simulink model "DiMauro_Galluzzi_Andres_2024_finalversion"  (R2024a)
settings: Solver=VariableStepAuto  StartTime=0.0  StopTime=simulation_time  RelTol=1e-3
values from neighbouring files (symbols this model uses):
  Ap = zeros(3)    [main.m]
  Bp = eye(3)    [main.m]
  degrad_flag = 1    [main.m]
  F = [e e e e e e; F_low]    [main.m]
  f_ex = 1    [main.m]
  g = 9.81    [main.m]
  Gamma_a = 0.001*eye(6)    [main.m]
  inv_M_tot = inv(M_tot)    [main.m]
  k_f = 3.65e-6    (= 3.65e-06)    [main.m]
  k_i_pos_control = K(3)    [main.m]
  k_omega = diag([K_w_x,K_w_y,K_w_z])    [main.m]
  k_p_pos_control = K(1)    [main.m]
  k_v_pos_control = K(2)    [main.m]
  L = 1    [main.m]
  lambda_r_0 = lambda_r*ones(6,1)    [main.m]
  M_tot = UAV.M+M_box    [main.m]
  omega_cmd_trim_1 = sqrt(UAV.m*g/(UAV.Nr*k_f))*[1 1 1 1 1 1]'    [main.m]
  omega_cmd_trim_2 = sqrt(T_rotor/k_f)*[1 1 1 1 1 1]'    [main.m]
  omega_r_0 = omega_cmd_trim_2    [main.m]
  omega_t = 0.1    [main.m]
  omegab_0 = [0 0 0]'    [main.m]
  p_0 = [0 0 1]'    [main.m]
  pert = 0*[1 1 1 0 0 0]'    [main.m]
  q_0 = eul2quat([0,theta_trim_2,0],'ZYX')'    [main.m]
  radius = 4    [main.m]
  t_pert = 50    [main.m]
  traj = 5    [main.m]
  trim_flag = 0    [main.m]
  vb_0 = 2*[cos(theta_trim_2) 0 sin(theta_trim_2)]'    [main.m]
  w_t = 1    [main.m]
undefined symbols (not defined in the file or in its folder): k_d_pos, k_i_velocity_control, UAV
libraries: slpidlib x6
settings Model: Creator=matti  LastModifiedBy=matti

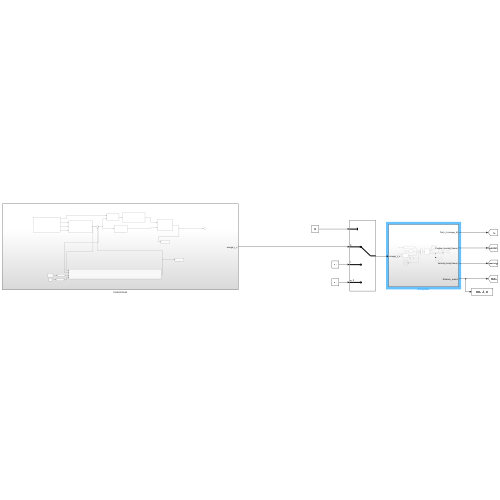
[thumbnail: Simulink's stored preview of the top-level diagram]
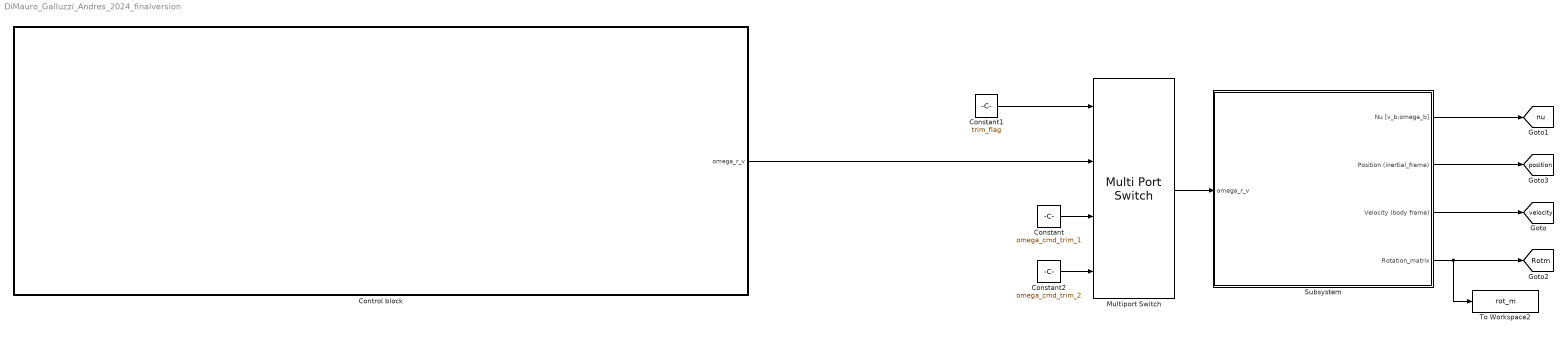
== system DiMauro_Galluzzi_Andres_2024_finalversion ==
  Constant : Constant  Value=omega_cmd_trim_1
  Constant1 : Constant  Value=trim_flag
  Constant2 : Constant  Value=omega_cmd_trim_2
  Control block : Subsystem
  Multiport Switch : MultiPortSwitch  DataPortOrder=Zero-based contiguous  zeroidx=on  SaturateOnIntegerOverflow=off  InputSameDT=off
  Subsystem : Subsystem
  To Workspace2 : ToWorkspace  VariableName=rot_m  SaveFormat=Timeseries  SampleTime=-1
  tag scope: Rotm=global, nu=global, position=global, velocity=global
  wires:
  Subsystem/1(Nu [v_b;omega_b]) -> [nu]
  Constant/1 -> Multiport Switch/3
  Constant2/1 -> Multiport Switch/4
  Subsystem/2(Position (inertial_frame)) -> [position]
  Subsystem/4(Rotation_matrix) -> To Workspace2/1, [Rotm]
  Subsystem/3(Velocity (body frame)) -> [velocity]
  Constant1/1 -> Multiport Switch/1
  Control block/1(omega_r_v) -> Multiport Switch/2
  Multiport Switch/1 -> Subsystem/1(omega_r_v)

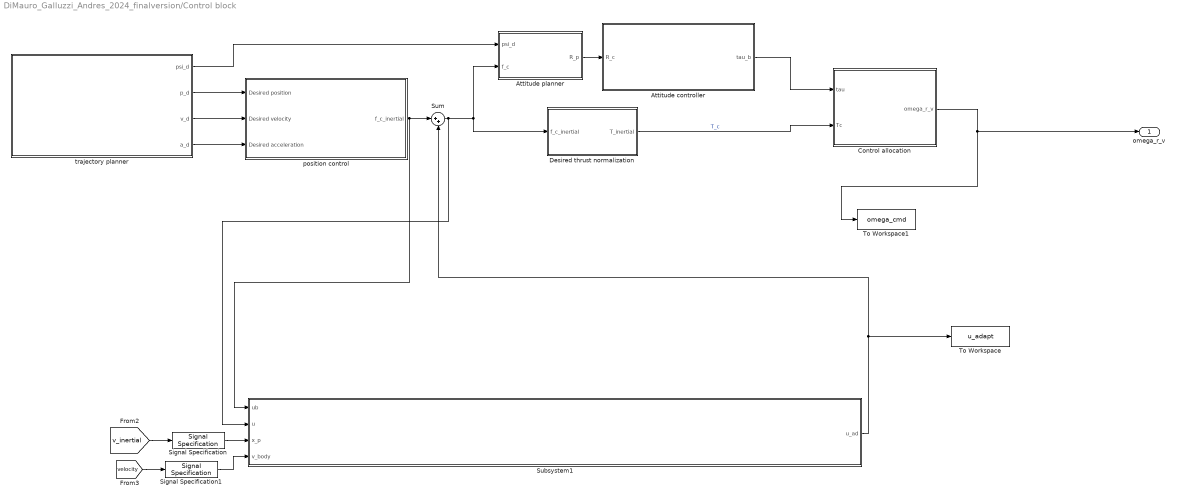
== system DiMauro_Galluzzi_Andres_2024_finalversion/Control block ==
  Attitude controller : Subsystem
  Attitude planner : MATLAB Function  TreatAsAtomicUnit=on
  Control allocation : MATLAB Function  TreatAsAtomicUnit=on
  Desired thrust normalization : MATLAB Function  TreatAsAtomicUnit=on
  Signal Specification : SignalSpecification  Dimensions=3
  Signal Specification1 : SignalSpecification  Dimensions=3
  Subsystem1 : Subsystem  Variant=on  AllowZeroVariantControls=on
  Sum : Sum  Inputs=|++
  To Workspace : ToWorkspace  VariableName=u_adapt  SaveFormat=Timeseries  SampleTime=-1
  To Workspace1 : ToWorkspace  VariableName=omega_cmd  SaveFormat=Timeseries  SampleTime=-1
  position control : Subsystem
  "trajectory planner " : Subsystem
  omega_r_v : Outport
  wires:
  Signal Specification/1 -> Subsystem1/3(x_p)
  Control allocation/1(omega_r_v) -> omega_r_v/1, To Workspace1/1
  Sum/1 -> Desired thrust normalization/1(f_c_inertial), Attitude planner/2(f_c), Subsystem1/2(u)
  Attitude planner/1(R_p) -> Attitude controller/1(R_c)
  [velocity] -> Signal Specification1/1
  Signal Specification1/1 -> Subsystem1/4(v_body)
  "trajectory planner "/1(psi_d) -> Attitude planner/1(psi_d)
  "trajectory planner "/2(p_d) -> position control/1(Desired position)
  [v_inertial] -> Signal Specification/1
  "trajectory planner "/3(v_d) -> position control/2(Desired velocity)
  Subsystem1/1(u_ad) -> To Workspace/1, Sum/2
  Desired thrust normalization/1(T_inertial) -> Control allocation/2(Tc)  "T_c"
  Attitude controller/1(tau_b) -> Control allocation/1(tau)
  "trajectory planner "/4(a_d) -> position control/3(Desired acceleration)
  position control/1(f_c_inertial) -> Sum/1, Subsystem1/1(ub)

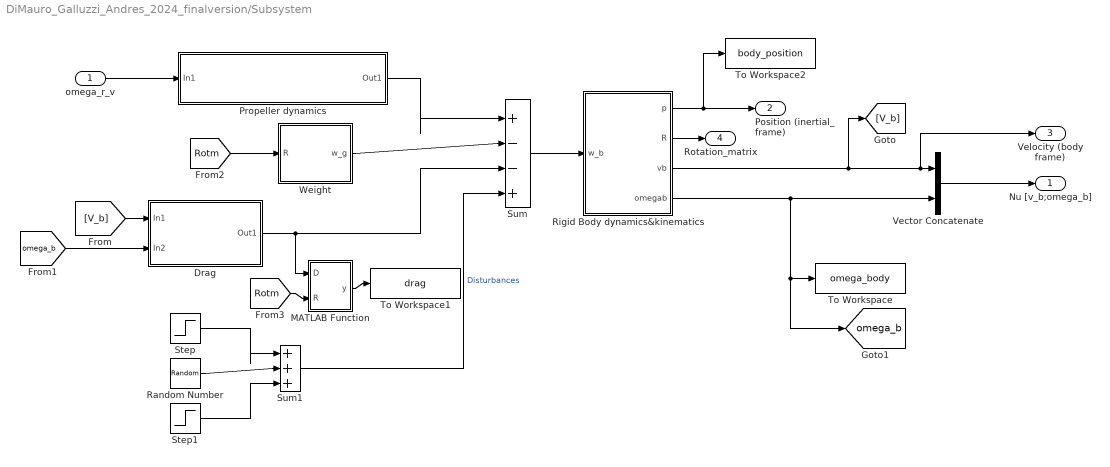
== system DiMauro_Galluzzi_Andres_2024_finalversion/Subsystem ==
  omega_r_v : Inport
  Drag : Subsystem
  MATLAB Function : MATLAB Function  TreatAsAtomicUnit=on
  Propeller dynamics : Subsystem
  Random Number : RandomNumber  Mean=[0 0 0 0 0 0]'  Variance=f_ex/20*[1 1 1 0 0 0]'  SampleTime=0.1
  "Rigid Body dynamics&kinematics " : Subsystem
  Step : Step  Time=t_pert  Before=0*[1 1 1 0 0 0]';  After=f_ex*[1 1 1 0 0 0]';  SampleTime=0
  Step1 : Step  Time=t_pert+5  Before=0*[1 1 1 0 0 0]';  After=-f_ex*[1 1 1 0 0 0]';  SampleTime=0
  Sum : Sum  Inputs=|+--+
  Sum1 : Sum  Inputs=|+++
  To Workspace : ToWorkspace  VariableName=omega_body  SaveFormat=Timeseries  SampleTime=-1
  To Workspace1 : ToWorkspace  VariableName=drag  SaveFormat=Timeseries  SampleTime=-1
  To Workspace2 : ToWorkspace  VariableName=body_position  SaveFormat=Timeseries  SampleTime=-1
  Vector Concatenate : Concatenate
  Weight : MATLAB Function  TreatAsAtomicUnit=on
  Nu [v_b;omega_b] : Outport
  Position (inertial_frame) : Outport  Port=2
  Velocity (body frame) : Outport  Port=3
  Rotation_matrix : Outport  Port=4
  tag scope: omega_b=global
  wires:
  "Rigid Body dynamics&kinematics "/3(vb) -> [V_b], Velocity (body frame)/1, Vector Concatenate/1
  [V_b] -> Drag/1(In1)
  "Rigid Body dynamics&kinematics "/4(omegab) -> [omega_b], To Workspace/1, Vector Concatenate/2
  Propeller dynamics/1(Out1) -> Sum/1
  Weight/1(w_g) -> Sum/2
  [Rotm] -> Weight/1(R)
  [omega_b] -> Drag/2(In2)
  Sum/1 -> "Rigid Body dynamics&kinematics "/1(w_b)
  omega_r_v/1 -> Propeller dynamics/1(In1)
  Vector Concatenate/1 -> Nu [v_b;omega_b]/1
  "Rigid Body dynamics&kinematics "/1(p) -> To Workspace2/1, Position (inertial_frame)/1
  "Rigid Body dynamics&kinematics "/2(R) -> Rotation_matrix/1
  Drag/1(Out1) -> MATLAB Function/1(D), Sum/3
  Random Number/1 -> Sum1/2
  Sum1/1 -> Sum/4  "Disturbances"
  Step/1 -> Sum1/1
  Step1/1 -> Sum1/3
  MATLAB Function/1(y) -> To Workspace1/1
  [Rotm] -> MATLAB Function/2(R)

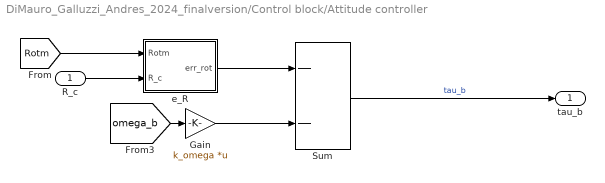
== system DiMauro_Galluzzi_Andres_2024_finalversion/Control block/Attitude controller ==
  R_c : Inport
  Gain : Gain  Gain=k_omega  Multiplication=Matrix(K*u)
  Sum : Sum  Inputs=--
  e_R : MATLAB Function  TreatAsAtomicUnit=on
  tau_b : Outport
  wires:
  e_R/1(err_rot) -> Sum/1
  [Rotm] -> e_R/1(Rotm)
  Sum/1 -> tau_b/1  "tau_b"
  [omega_b] -> Gain/1
  R_c/1 -> e_R/2(R_c)
  Gain/1 -> Sum/2

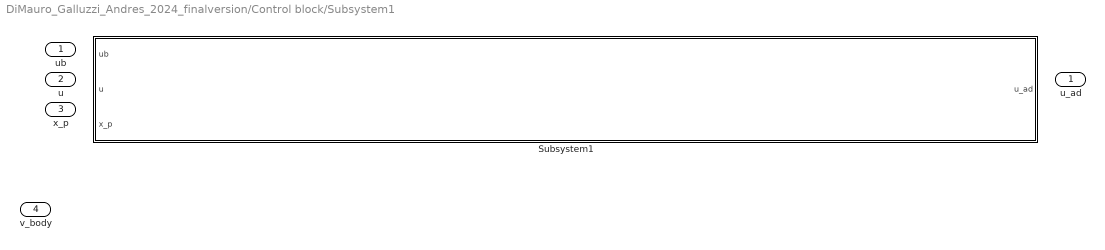
== system DiMauro_Galluzzi_Andres_2024_finalversion/Control block/Subsystem1 ==
  ub : Inport
  u : Inport  Port=2
  x_p : Inport  Port=3
  v_body : Inport  Port=4
  Subsystem1 : Subsystem  VariantControl=flag_adaptive==1
  u_ad : Outport

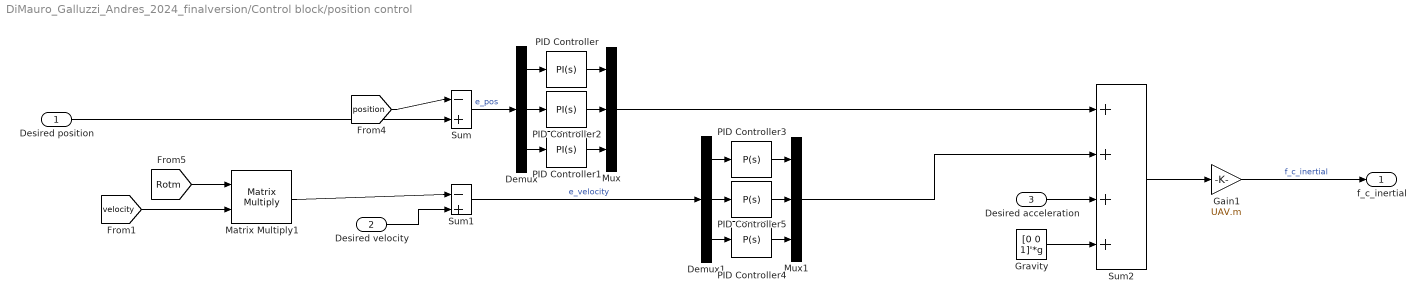
== system DiMauro_Galluzzi_Andres_2024_finalversion/Control block/position control ==
  Desired position : Inport
  Desired velocity : Inport  Port=2
  Desired acceleration : Inport  Port=3
  Demux : Demux  Outputs=3
  Demux1 : Demux  Outputs=3
  Gain1 : Gain  Gain=UAV.m
  Gravity : Constant  Value=[0 0 1]'*g
  Matrix Multiply1 : Product  Multiplication=Matrix(*)
  Mux : Mux  Inputs=3
  Mux1 : Mux  Inputs=3
  PID Controller : slpidlib/PID Controller  Controller=PI  Form=Parallel  TimeDomain=Continuous-time  UseExternalTs=off  SampleTime=-1  IntegratorMethod=Forward Euler  FilterMethod=Forward Euler  ControllerParametersSource=internal  P=k_p_pos_control  I=k_i_pos_control  UseKiTs=off  D=k_d_pos  UseExternalDerivativeSource=off  N=100  UseFilter=on  TunerSelectOption=Transfer Function Based (PID Tuner App)  InitialConditionSource=internal  InitialConditionForIntegrator=0  InitialConditionForFilter=0  DifferentiatorICPrevScaledInput=0  ExternalReset=none  TrackingMode=off  Kt=1  LimitOutput=off  SatLimitsSource=internal  UpperSaturationLimit=inf  LowerSaturationLimit=-inf  LinearizeAsGain=on  AntiWindupMode=none  Kb=1  LimitIntegrator=off  UpperIntegratorSaturationLimit=inf  LowerIntegratorSaturationLimit=-inf  POutMin=[]  POutMax=[]  IOutMin=[]  IOutMax=[]  DOutMin=[]  DOutMax=[]  NOutMin=[]  NOutMax=[]  SumOutMin=[]  SumOutMax=[]  SaturationOutMin=[]  SaturationOutMax=[]  PParamMin=[]  PParamMax=[]  IParamMin=[]  IParamMax=[]  DParamMin=[]  DParamMax=[]  NParamMin=[]  NParamMax=[]  KbParamMin=[]  KbParamMax=[]  KtParamMin=[]  KtParamMax=[]  KbOutMin=[]  KbOutMax=[]  KtOutMin=[]  KtOutMax=[]  IntegratorOutMin=[]  IntegratorOutMax=[]  FilterOutMin=[]  FilterOutMax=[]  SumI1OutMin=[]  SumI1OutMax=[]  SumI2OutMin=[]  SumI2OutMax=[]  SumI3OutMin=[]  SumI3OutMax=[]  SumI4OutMin=[]  SumI4OutMax=[]  SumDOutMin=[]  SumDOutMax=[]  DifferentiatorOutMin=[]  DifferentiatorOutMax=[]  FilterDiffOutCoefMin=[]  FilterDiffOutCoefMax=[]  ReciprocalOutMin=[]  ReciprocalOutMax=[]  SumDenOutMin=[]  SumDenOutMax=[]  SumNumOutMin=[]  SumNumOutMax=[]  DivideOutMin=[]  DivideOutMax=[]  UdiffTsProdOutMin=[]  UdiffTsProdOutMax=[]  NTsProdOutMin=[]  NTsProdOutMax=[]  UintegralTsProdOutMin=[]  UintegralTsProdOutMax=[]  UngainTsProdOutMin=[]  UngainTsProdOutMax=[]  ClampingZeroOutDataTypeStr=Inherit: Inherit via back propagation  ClampingZeroOutMin=[]  ClampingZeroOutMax=[]  FilterDenConstantOutDataTypeStr=Inherit: Inherit via back propagation  FilterDenConstantOutMin=[]  FilterDenConstantOutMax=[]  PCopyOutDataTypeStr=Inherit: Inherit via back propagation  PCopyOutMin=[]  PCopyOutMax=[]  NCopyOutDataTypeStr=Inherit: Inherit via back propagation  NCopyOutMin=[]  NCopyOutMax=[]  IntegratorContinuousStateAttributes=''  IntegratorStateMustResolveToSignalObject=off  IntegratorRTWStateStorageClass=Auto  FilterContinuousStateAttributes=''  FilterStateMustResolveToSignalObject=off  FilterRTWStateStorageClass=Auto  ParallelPVariant=InternalParameters  IdealPVariant=Disabled  IVariant=InternalParameters  DVariant=Disabled  IntegratorVariant=Continuous  SatVariant=Disabled  AWVariant=Passthrough  PCopyVariant=Disabled  TRVariant=Disabled  FdbkBlocksVariant=Forward  IdealPFdbkVariant=Disabled  SatFdbkVariant=Disabled  DerivativeFilterVariant=Disabled  NVariant=Disabled  NCopyVariant=Disabled_SignalSpec  FilterICVariant=Disabled  IntegratorICVariant=InternalICs  ExternalResetVariant=Disabled  TRSumVariant=Passthrough  SumFdbkVariant=Disabled  SumVariant=Sum_PI  TsampFilterVariant=InternalTs  TsampNgainVariant=Passthrough  TsampIntegralVariant=Disabled_SignalSpec  ExternalSaturationOutDataTypeStr=Inherit: Same as second input  DerivativeSourceVariant=Disabled
  PID Controller1 : slpidlib/PID Controller  Controller=PI  Form=Parallel  TimeDomain=Continuous-time  UseExternalTs=off  SampleTime=-1  IntegratorMethod=Forward Euler  FilterMethod=Forward Euler  ControllerParametersSource=internal  P=k_p_pos_control  I=k_i_pos_control  UseKiTs=off  D=k_d_pos  UseExternalDerivativeSource=off  N=100  UseFilter=on  TunerSelectOption=Transfer Function Based (PID Tuner App)  InitialConditionSource=internal  InitialConditionForIntegrator=0  InitialConditionForFilter=0  DifferentiatorICPrevScaledInput=0  ExternalReset=none  TrackingMode=off  Kt=1  LimitOutput=off  SatLimitsSource=internal  UpperSaturationLimit=inf  LowerSaturationLimit=-inf  LinearizeAsGain=on  AntiWindupMode=none  Kb=1  LimitIntegrator=off  UpperIntegratorSaturationLimit=inf  LowerIntegratorSaturationLimit=-inf  POutMin=[]  POutMax=[]  IOutMin=[]  IOutMax=[]  DOutMin=[]  DOutMax=[]  NOutMin=[]  NOutMax=[]  SumOutMin=[]  SumOutMax=[]  SaturationOutMin=[]  SaturationOutMax=[]  PParamMin=[]  PParamMax=[]  IParamMin=[]  IParamMax=[]  DParamMin=[]  DParamMax=[]  NParamMin=[]  NParamMax=[]  KbParamMin=[]  KbParamMax=[]  KtParamMin=[]  KtParamMax=[]  KbOutMin=[]  KbOutMax=[]  KtOutMin=[]  KtOutMax=[]  IntegratorOutMin=[]  IntegratorOutMax=[]  FilterOutMin=[]  FilterOutMax=[]  SumI1OutMin=[]  SumI1OutMax=[]  SumI2OutMin=[]  SumI2OutMax=[]  SumI3OutMin=[]  SumI3OutMax=[]  SumI4OutMin=[]  SumI4OutMax=[]  SumDOutMin=[]  SumDOutMax=[]  DifferentiatorOutMin=[]  DifferentiatorOutMax=[]  FilterDiffOutCoefMin=[]  FilterDiffOutCoefMax=[]  ReciprocalOutMin=[]  ReciprocalOutMax=[]  SumDenOutMin=[]  SumDenOutMax=[]  SumNumOutMin=[]  SumNumOutMax=[]  DivideOutMin=[]  DivideOutMax=[]  UdiffTsProdOutMin=[]  UdiffTsProdOutMax=[]  NTsProdOutMin=[]  NTsProdOutMax=[]  UintegralTsProdOutMin=[]  UintegralTsProdOutMax=[]  UngainTsProdOutMin=[]  UngainTsProdOutMax=[]  ClampingZeroOutDataTypeStr=Inherit: Inherit via back propagation  ClampingZeroOutMin=[]  ClampingZeroOutMax=[]  FilterDenConstantOutDataTypeStr=Inherit: Inherit via back propagation  FilterDenConstantOutMin=[]  FilterDenConstantOutMax=[]  PCopyOutDataTypeStr=Inherit: Inherit via back propagation  PCopyOutMin=[]  PCopyOutMax=[]  NCopyOutDataTypeStr=Inherit: Inherit via back propagation  NCopyOutMin=[]  NCopyOutMax=[]  IntegratorContinuousStateAttributes=''  IntegratorStateMustResolveToSignalObject=off  IntegratorRTWStateStorageClass=Auto  FilterContinuousStateAttributes=''  FilterStateMustResolveToSignalObject=off  FilterRTWStateStorageClass=Auto  ParallelPVariant=InternalParameters  IdealPVariant=Disabled  IVariant=InternalParameters  DVariant=Disabled  IntegratorVariant=Continuous  SatVariant=Disabled  AWVariant=Passthrough  PCopyVariant=Disabled  TRVariant=Disabled  FdbkBlocksVariant=Forward  IdealPFdbkVariant=Disabled  SatFdbkVariant=Disabled  DerivativeFilterVariant=Disabled  NVariant=Disabled  NCopyVariant=Disabled_SignalSpec  FilterICVariant=Disabled  IntegratorICVariant=InternalICs  ExternalResetVariant=Disabled  TRSumVariant=Passthrough  SumFdbkVariant=Disabled  SumVariant=Sum_PI  TsampFilterVariant=InternalTs  TsampNgainVariant=Passthrough  TsampIntegralVariant=Disabled_SignalSpec  ExternalSaturationOutDataTypeStr=Inherit: Same as second input  DerivativeSourceVariant=Disabled
  PID Controller2 : slpidlib/PID Controller  Controller=PI  Form=Parallel  TimeDomain=Continuous-time  UseExternalTs=off  SampleTime=-1  IntegratorMethod=Forward Euler  FilterMethod=Forward Euler  ControllerParametersSource=internal  P=k_p_pos_control  I=k_i_pos_control  UseKiTs=off  D=k_d_pos  UseExternalDerivativeSource=off  N=100  UseFilter=on  TunerSelectOption=Transfer Function Based (PID Tuner App)  InitialConditionSource=internal  InitialConditionForIntegrator=0  InitialConditionForFilter=0  DifferentiatorICPrevScaledInput=0  ExternalReset=none  TrackingMode=off  Kt=1  LimitOutput=off  SatLimitsSource=internal  UpperSaturationLimit=inf  LowerSaturationLimit=-inf  LinearizeAsGain=on  AntiWindupMode=none  Kb=1  LimitIntegrator=off  UpperIntegratorSaturationLimit=inf  LowerIntegratorSaturationLimit=-inf  POutMin=[]  POutMax=[]  IOutMin=[]  IOutMax=[]  DOutMin=[]  DOutMax=[]  NOutMin=[]  NOutMax=[]  SumOutMin=[]  SumOutMax=[]  SaturationOutMin=[]  SaturationOutMax=[]  PParamMin=[]  PParamMax=[]  IParamMin=[]  IParamMax=[]  DParamMin=[]  DParamMax=[]  NParamMin=[]  NParamMax=[]  KbParamMin=[]  KbParamMax=[]  KtParamMin=[]  KtParamMax=[]  KbOutMin=[]  KbOutMax=[]  KtOutMin=[]  KtOutMax=[]  IntegratorOutMin=[]  IntegratorOutMax=[]  FilterOutMin=[]  FilterOutMax=[]  SumI1OutMin=[]  SumI1OutMax=[]  SumI2OutMin=[]  SumI2OutMax=[]  SumI3OutMin=[]  SumI3OutMax=[]  SumI4OutMin=[]  SumI4OutMax=[]  SumDOutMin=[]  SumDOutMax=[]  DifferentiatorOutMin=[]  DifferentiatorOutMax=[]  FilterDiffOutCoefMin=[]  FilterDiffOutCoefMax=[]  ReciprocalOutMin=[]  ReciprocalOutMax=[]  SumDenOutMin=[]  SumDenOutMax=[]  SumNumOutMin=[]  SumNumOutMax=[]  DivideOutMin=[]  DivideOutMax=[]  UdiffTsProdOutMin=[]  UdiffTsProdOutMax=[]  NTsProdOutMin=[]  NTsProdOutMax=[]  UintegralTsProdOutMin=[]  UintegralTsProdOutMax=[]  UngainTsProdOutMin=[]  UngainTsProdOutMax=[]  ClampingZeroOutDataTypeStr=Inherit: Inherit via back propagation  ClampingZeroOutMin=[]  ClampingZeroOutMax=[]  FilterDenConstantOutDataTypeStr=Inherit: Inherit via back propagation  FilterDenConstantOutMin=[]  FilterDenConstantOutMax=[]  PCopyOutDataTypeStr=Inherit: Inherit via back propagation  PCopyOutMin=[]  PCopyOutMax=[]  NCopyOutDataTypeStr=Inherit: Inherit via back propagation  NCopyOutMin=[]  NCopyOutMax=[]  IntegratorContinuousStateAttributes=''  IntegratorStateMustResolveToSignalObject=off  IntegratorRTWStateStorageClass=Auto  FilterContinuousStateAttributes=''  FilterStateMustResolveToSignalObject=off  FilterRTWStateStorageClass=Auto  ParallelPVariant=InternalParameters  IdealPVariant=Disabled  IVariant=InternalParameters  DVariant=Disabled  IntegratorVariant=Continuous  SatVariant=Disabled  AWVariant=Passthrough  PCopyVariant=Disabled  TRVariant=Disabled  FdbkBlocksVariant=Forward  IdealPFdbkVariant=Disabled  SatFdbkVariant=Disabled  DerivativeFilterVariant=Disabled  NVariant=Disabled  NCopyVariant=Disabled_SignalSpec  FilterICVariant=Disabled  IntegratorICVariant=InternalICs  ExternalResetVariant=Disabled  TRSumVariant=Passthrough  SumFdbkVariant=Disabled  SumVariant=Sum_PI  TsampFilterVariant=InternalTs  TsampNgainVariant=Passthrough  TsampIntegralVariant=Disabled_SignalSpec  ExternalSaturationOutDataTypeStr=Inherit: Same as second input  DerivativeSourceVariant=Disabled
  PID Controller3 : slpidlib/PID Controller  Controller=P  Form=Parallel  TimeDomain=Continuous-time  UseExternalTs=off  SampleTime=-1  IntegratorMethod=Forward Euler  FilterMethod=Forward Euler  ControllerParametersSource=internal  P=k_v_pos_control  I=k_i_velocity_control  UseKiTs=off  D=0  UseExternalDerivativeSource=off  N=100  UseFilter=on  TunerSelectOption=Transfer Function Based (PID Tuner App)  InitialConditionSource=internal  InitialConditionForIntegrator=0  InitialConditionForFilter=0  DifferentiatorICPrevScaledInput=0  ExternalReset=none  TrackingMode=off  Kt=1  LimitOutput=off  SatLimitsSource=internal  UpperSaturationLimit=inf  LowerSaturationLimit=-inf  LinearizeAsGain=on  AntiWindupMode=none  Kb=1  LimitIntegrator=off  UpperIntegratorSaturationLimit=inf  LowerIntegratorSaturationLimit=-inf  POutMin=[]  POutMax=[]  IOutMin=[]  IOutMax=[]  DOutMin=[]  DOutMax=[]  NOutMin=[]  NOutMax=[]  SumOutMin=[]  SumOutMax=[]  SaturationOutMin=[]  SaturationOutMax=[]  PParamMin=[]  PParamMax=[]  IParamMin=[]  IParamMax=[]  DParamMin=[]  DParamMax=[]  NParamMin=[]  NParamMax=[]  KbParamMin=[]  KbParamMax=[]  KtParamMin=[]  KtParamMax=[]  KbOutMin=[]  KbOutMax=[]  KtOutMin=[]  KtOutMax=[]  IntegratorOutMin=[]  IntegratorOutMax=[]  FilterOutMin=[]  FilterOutMax=[]  SumI1OutMin=[]  SumI1OutMax=[]  SumI2OutMin=[]  SumI2OutMax=[]  SumI3OutMin=[]  SumI3OutMax=[]  SumI4OutMin=[]  SumI4OutMax=[]  SumDOutMin=[]  SumDOutMax=[]  DifferentiatorOutMin=[]  DifferentiatorOutMax=[]  FilterDiffOutCoefMin=[]  FilterDiffOutCoefMax=[]  ReciprocalOutMin=[]  ReciprocalOutMax=[]  SumDenOutMin=[]  SumDenOutMax=[]  SumNumOutMin=[]  SumNumOutMax=[]  DivideOutMin=[]  DivideOutMax=[]  UdiffTsProdOutMin=[]  UdiffTsProdOutMax=[]  NTsProdOutMin=[]  NTsProdOutMax=[]  UintegralTsProdOutMin=[]  UintegralTsProdOutMax=[]  UngainTsProdOutMin=[]  UngainTsProdOutMax=[]  ClampingZeroOutDataTypeStr=Inherit: Inherit via back propagation  ClampingZeroOutMin=[]  ClampingZeroOutMax=[]  FilterDenConstantOutDataTypeStr=Inherit: Inherit via back propagation  FilterDenConstantOutMin=[]  FilterDenConstantOutMax=[]  PCopyOutDataTypeStr=Inherit: Inherit via back propagation  PCopyOutMin=[]  PCopyOutMax=[]  NCopyOutDataTypeStr=Inherit: Inherit via back propagation  NCopyOutMin=[]  NCopyOutMax=[]  IntegratorContinuousStateAttributes=''  IntegratorStateMustResolveToSignalObject=off  IntegratorRTWStateStorageClass=Auto  FilterContinuousStateAttributes=''  FilterStateMustResolveToSignalObject=off  FilterRTWStateStorageClass=Auto  ParallelPVariant=InternalParameters  IdealPVariant=Disabled  IVariant=Disabled  DVariant=Disabled  IntegratorVariant=Disabled  SatVariant=Disabled  AWVariant=Disabled  PCopyVariant=Disabled  TRVariant=Disabled  FdbkBlocksVariant=Forward  IdealPFdbkVariant=Disabled  SatFdbkVariant=Disabled  DerivativeFilterVariant=Disabled  NVariant=Disabled  NCopyVariant=Disabled_SignalSpec  FilterICVariant=Disabled  IntegratorICVariant=Disabled  ExternalResetVariant=Disabled  TRSumVariant=Passthrough  SumFdbkVariant=Disabled  SumVariant=Passthrough_P  TsampFilterVariant=InternalTs  TsampNgainVariant=Passthrough  TsampIntegralVariant=Disabled_SignalSpec  ExternalSaturationOutDataTypeStr=Inherit: Same as second input  DerivativeSourceVariant=Disabled
  PID Controller4 : slpidlib/PID Controller  Controller=P  Form=Parallel  TimeDomain=Continuous-time  UseExternalTs=off  SampleTime=-1  IntegratorMethod=Forward Euler  FilterMethod=Forward Euler  ControllerParametersSource=internal  P=k_v_pos_control  I=k_i_velocity_control*5  UseKiTs=off  D=0  UseExternalDerivativeSource=off  N=100  UseFilter=on  TunerSelectOption=Transfer Function Based (PID Tuner App)  InitialConditionSource=internal  InitialConditionForIntegrator=0  InitialConditionForFilter=0  DifferentiatorICPrevScaledInput=0  ExternalReset=none  TrackingMode=off  Kt=1  LimitOutput=off  SatLimitsSource=internal  UpperSaturationLimit=inf  LowerSaturationLimit=-inf  LinearizeAsGain=on  AntiWindupMode=none  Kb=1  LimitIntegrator=off  UpperIntegratorSaturationLimit=inf  LowerIntegratorSaturationLimit=-inf  POutMin=[]  POutMax=[]  IOutMin=[]  IOutMax=[]  DOutMin=[]  DOutMax=[]  NOutMin=[]  NOutMax=[]  SumOutMin=[]  SumOutMax=[]  SaturationOutMin=[]  SaturationOutMax=[]  PParamMin=[]  PParamMax=[]  IParamMin=[]  IParamMax=[]  DParamMin=[]  DParamMax=[]  NParamMin=[]  NParamMax=[]  KbParamMin=[]  KbParamMax=[]  KtParamMin=[]  KtParamMax=[]  KbOutMin=[]  KbOutMax=[]  KtOutMin=[]  KtOutMax=[]  IntegratorOutMin=[]  IntegratorOutMax=[]  FilterOutMin=[]  FilterOutMax=[]  SumI1OutMin=[]  SumI1OutMax=[]  SumI2OutMin=[]  SumI2OutMax=[]  SumI3OutMin=[]  SumI3OutMax=[]  SumI4OutMin=[]  SumI4OutMax=[]  SumDOutMin=[]  SumDOutMax=[]  DifferentiatorOutMin=[]  DifferentiatorOutMax=[]  FilterDiffOutCoefMin=[]  FilterDiffOutCoefMax=[]  ReciprocalOutMin=[]  ReciprocalOutMax=[]  SumDenOutMin=[]  SumDenOutMax=[]  SumNumOutMin=[]  SumNumOutMax=[]  DivideOutMin=[]  DivideOutMax=[]  UdiffTsProdOutMin=[]  UdiffTsProdOutMax=[]  NTsProdOutMin=[]  NTsProdOutMax=[]  UintegralTsProdOutMin=[]  UintegralTsProdOutMax=[]  UngainTsProdOutMin=[]  UngainTsProdOutMax=[]  ClampingZeroOutDataTypeStr=Inherit: Inherit via back propagation  ClampingZeroOutMin=[]  ClampingZeroOutMax=[]  FilterDenConstantOutDataTypeStr=Inherit: Inherit via back propagation  FilterDenConstantOutMin=[]  FilterDenConstantOutMax=[]  PCopyOutDataTypeStr=Inherit: Inherit via back propagation  PCopyOutMin=[]  PCopyOutMax=[]  NCopyOutDataTypeStr=Inherit: Inherit via back propagation  NCopyOutMin=[]  NCopyOutMax=[]  IntegratorContinuousStateAttributes=''  IntegratorStateMustResolveToSignalObject=off  IntegratorRTWStateStorageClass=Auto  FilterContinuousStateAttributes=''  FilterStateMustResolveToSignalObject=off  FilterRTWStateStorageClass=Auto  ParallelPVariant=InternalParameters  IdealPVariant=Disabled  IVariant=Disabled  DVariant=Disabled  IntegratorVariant=Disabled  SatVariant=Disabled  AWVariant=Disabled  PCopyVariant=Disabled  TRVariant=Disabled  FdbkBlocksVariant=Forward  IdealPFdbkVariant=Disabled  SatFdbkVariant=Disabled  DerivativeFilterVariant=Disabled  NVariant=Disabled  NCopyVariant=Disabled_SignalSpec  FilterICVariant=Disabled  IntegratorICVariant=Disabled  ExternalResetVariant=Disabled  TRSumVariant=Passthrough  SumFdbkVariant=Disabled  SumVariant=Passthrough_P  TsampFilterVariant=InternalTs  TsampNgainVariant=Passthrough  TsampIntegralVariant=Disabled_SignalSpec  ExternalSaturationOutDataTypeStr=Inherit: Same as second input  DerivativeSourceVariant=Disabled
  PID Controller5 : slpidlib/PID Controller  Controller=P  Form=Parallel  TimeDomain=Continuous-time  UseExternalTs=off  SampleTime=-1  IntegratorMethod=Forward Euler  FilterMethod=Forward Euler  ControllerParametersSource=internal  P=k_v_pos_control  I=k_i_velocity_control  UseKiTs=off  D=0  UseExternalDerivativeSource=off  N=100  UseFilter=on  TunerSelectOption=Transfer Function Based (PID Tuner App)  InitialConditionSource=internal  InitialConditionForIntegrator=0  InitialConditionForFilter=0  DifferentiatorICPrevScaledInput=0  ExternalReset=none  TrackingMode=off  Kt=1  LimitOutput=off  SatLimitsSource=internal  UpperSaturationLimit=inf  LowerSaturationLimit=-inf  LinearizeAsGain=on  AntiWindupMode=none  Kb=1  LimitIntegrator=off  UpperIntegratorSaturationLimit=inf  LowerIntegratorSaturationLimit=-inf  POutMin=[]  POutMax=[]  IOutMin=[]  IOutMax=[]  DOutMin=[]  DOutMax=[]  NOutMin=[]  NOutMax=[]  SumOutMin=[]  SumOutMax=[]  SaturationOutMin=[]  SaturationOutMax=[]  PParamMin=[]  PParamMax=[]  IParamMin=[]  IParamMax=[]  DParamMin=[]  DParamMax=[]  NParamMin=[]  NParamMax=[]  KbParamMin=[]  KbParamMax=[]  KtParamMin=[]  KtParamMax=[]  KbOutMin=[]  KbOutMax=[]  KtOutMin=[]  KtOutMax=[]  IntegratorOutMin=[]  IntegratorOutMax=[]  FilterOutMin=[]  FilterOutMax=[]  SumI1OutMin=[]  SumI1OutMax=[]  SumI2OutMin=[]  SumI2OutMax=[]  SumI3OutMin=[]  SumI3OutMax=[]  SumI4OutMin=[]  SumI4OutMax=[]  SumDOutMin=[]  SumDOutMax=[]  DifferentiatorOutMin=[]  DifferentiatorOutMax=[]  FilterDiffOutCoefMin=[]  FilterDiffOutCoefMax=[]  ReciprocalOutMin=[]  ReciprocalOutMax=[]  SumDenOutMin=[]  SumDenOutMax=[]  SumNumOutMin=[]  SumNumOutMax=[]  DivideOutMin=[]  DivideOutMax=[]  UdiffTsProdOutMin=[]  UdiffTsProdOutMax=[]  NTsProdOutMin=[]  NTsProdOutMax=[]  UintegralTsProdOutMin=[]  UintegralTsProdOutMax=[]  UngainTsProdOutMin=[]  UngainTsProdOutMax=[]  ClampingZeroOutDataTypeStr=Inherit: Inherit via back propagation  ClampingZeroOutMin=[]  ClampingZeroOutMax=[]  FilterDenConstantOutDataTypeStr=Inherit: Inherit via back propagation  FilterDenConstantOutMin=[]  FilterDenConstantOutMax=[]  PCopyOutDataTypeStr=Inherit: Inherit via back propagation  PCopyOutMin=[]  PCopyOutMax=[]  NCopyOutDataTypeStr=Inherit: Inherit via back propagation  NCopyOutMin=[]  NCopyOutMax=[]  IntegratorContinuousStateAttributes=''  IntegratorStateMustResolveToSignalObject=off  IntegratorRTWStateStorageClass=Auto  FilterContinuousStateAttributes=''  FilterStateMustResolveToSignalObject=off  FilterRTWStateStorageClass=Auto  ParallelPVariant=InternalParameters  IdealPVariant=Disabled  IVariant=Disabled  DVariant=Disabled  IntegratorVariant=Disabled  SatVariant=Disabled  AWVariant=Disabled  PCopyVariant=Disabled  TRVariant=Disabled  FdbkBlocksVariant=Forward  IdealPFdbkVariant=Disabled  SatFdbkVariant=Disabled  DerivativeFilterVariant=Disabled  NVariant=Disabled  NCopyVariant=Disabled_SignalSpec  FilterICVariant=Disabled  IntegratorICVariant=Disabled  ExternalResetVariant=Disabled  TRSumVariant=Passthrough  SumFdbkVariant=Disabled  SumVariant=Passthrough_P  TsampFilterVariant=InternalTs  TsampNgainVariant=Passthrough  TsampIntegralVariant=Disabled_SignalSpec  ExternalSaturationOutDataTypeStr=Inherit: Same as second input  DerivativeSourceVariant=Disabled
  Sum : Sum  Inputs=|-+
  Sum1 : Sum  Inputs=|-+
  Sum2 : Sum  Inputs=++++
  f_c_inertial : Outport
  wires:
  Sum2/1 -> Gain1/1
  [position] -> Sum/1
  Gravity/1 -> Sum2/4
  Desired velocity/1 -> Sum1/2
  Desired acceleration/1 -> Sum2/3
  Desired position/1 -> Sum/2
  [velocity] -> Matrix Multiply1/2
  Matrix Multiply1/1 -> Sum1/1
  [Rotm] -> Matrix Multiply1/1
  Gain1/1 -> f_c_inertial/1  "f_c_inertial"
  Sum/1 -> Demux/1  "e_pos"
  Demux/2 -> PID Controller2/1
  Demux/3 -> PID Controller1/1
  PID Controller2/1 -> Mux/2
  PID Controller/1 -> Mux/1
  PID Controller1/1 -> Mux/3
  Demux/1 -> PID Controller/1
  Demux1/3 -> PID Controller4/1
  PID Controller3/1 -> Mux1/1
  PID Controller5/1 -> Mux1/2
  PID Controller4/1 -> Mux1/3
  Demux1/2 -> PID Controller5/1
  Demux1/1 -> PID Controller3/1
  Mux1/1 -> Sum2/2
  Sum1/1 -> Demux1/1  "e_velocity"
  Mux/1 -> Sum2/1

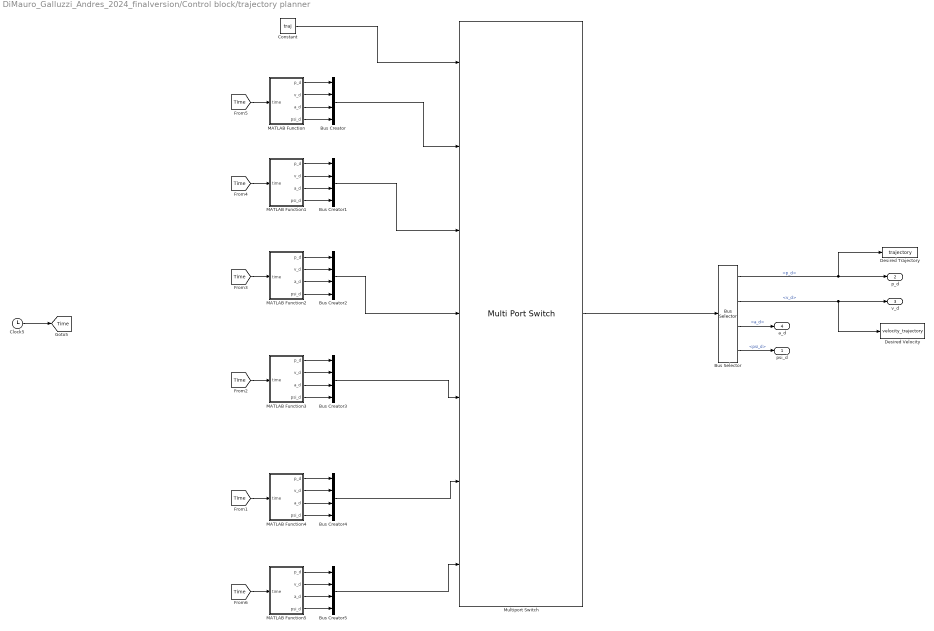
== system DiMauro_Galluzzi_Andres_2024_finalversion/Control block/trajectory planner  ==
  Bus Creator{,1..5} (6 alike) : BusCreator  Inputs=4
  Bus Selector : BusSelector  OutputSignals=p_d,v_d,a_d,psi_d
  Clock5 : Clock
  Constant : Constant  Value=traj
  Desired Trajectory : ToWorkspace  VariableName=trajectory  SaveFormat=Timeseries  SampleTime=-1
  Desired Velocity : ToWorkspace  VariableName=velocity_trajectory  SaveFormat=Timeseries  SampleTime=-1
  MATLAB Function : MATLAB Function  TreatAsAtomicUnit=on
  MATLAB Function1 : MATLAB Function  TreatAsAtomicUnit=on
  MATLAB Function2 : MATLAB Function  TreatAsAtomicUnit=on
  MATLAB Function3 : MATLAB Function  TreatAsAtomicUnit=on
  MATLAB Function4 : MATLAB Function  TreatAsAtomicUnit=on
  MATLAB Function5 : MATLAB Function  TreatAsAtomicUnit=on
  Multiport Switch : MultiPortSwitch  DataPortOrder=Zero-based contiguous  Inputs=6  zeroidx=on  SaturateOnIntegerOverflow=off  InputSameDT=off
  psi_d : Outport
  p_d : Outport  Port=2
  v_d : Outport  Port=3
  a_d : Outport  Port=4
  tag scope: Time=global
  wires:
  Constant/1 -> Multiport Switch/1
  Bus Creator/1 -> Multiport Switch/2
  MATLAB Function/1(p_d) -> Bus Creator/1
  MATLAB Function/2(v_d) -> Bus Creator/2
  MATLAB Function/3(a_d) -> Bus Creator/3
  MATLAB Function/4(psi_d) -> Bus Creator/4
  MATLAB Function1/4(psi_d) -> Bus Creator1/4
  MATLAB Function1/1(p_d) -> Bus Creator1/1
  Bus Creator1/1 -> Multiport Switch/3
  MATLAB Function1/3(a_d) -> Bus Creator1/3
  MATLAB Function1/2(v_d) -> Bus Creator1/2
  MATLAB Function2/4(psi_d) -> Bus Creator2/4
  MATLAB Function2/1(p_d) -> Bus Creator2/1
  Bus Creator2/1 -> Multiport Switch/4
  MATLAB Function2/3(a_d) -> Bus Creator2/3
  MATLAB Function2/2(v_d) -> Bus Creator2/2
  MATLAB Function3/4(psi_d) -> Bus Creator3/4
  MATLAB Function3/1(p_d) -> Bus Creator3/1
  Bus Creator3/1 -> Multiport Switch/5
  MATLAB Function3/3(a_d) -> Bus Creator3/3
  MATLAB Function3/2(v_d) -> Bus Creator3/2
  Multiport Switch/1 -> Bus Selector/1
  Bus Selector/4 -> psi_d/1  "<psi_d>"
  Bus Selector/3 -> a_d/1  "<a_d>"
  Bus Selector/2 -> Desired Velocity/1, v_d/1  "<v_d>"
  Bus Selector/1 -> Desired Trajectory/1, p_d/1  "<p_d>"
  MATLAB Function4/3(a_d) -> Bus Creator4/3
  MATLAB Function4/2(v_d) -> Bus Creator4/2
  MATLAB Function4/1(p_d) -> Bus Creator4/1
  MATLAB Function4/4(psi_d) -> Bus Creator4/4
  Bus Creator4/1 -> Multiport Switch/6
  Clock5/1 -> [Time]
  [Time] -> MATLAB Function/1(time)
  [Time] -> MATLAB Function1/1(time)
  [Time] -> MATLAB Function2/1(time)
  [Time] -> MATLAB Function3/1(time)
  [Time] -> MATLAB Function4/1(time)
  MATLAB Function5/2(v_d) -> Bus Creator5/2
  MATLAB Function5/4(psi_d) -> Bus Creator5/4
  Bus Creator5/1 -> Multiport Switch/7
  [Time] -> MATLAB Function5/1(time)
  MATLAB Function5/1(p_d) -> Bus Creator5/1
  MATLAB Function5/3(a_d) -> Bus Creator5/3

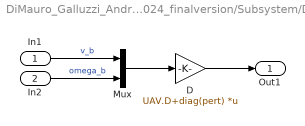
== system DiMauro_Galluzzi_Andres_2024_finalversion/Subsystem/Drag ==
  In1 : Inport
  In2 : Inport  Port=2
  D : Gain  Gain=UAV.D+diag(pert)  Multiplication=Matrix(K*u)
  Mux : Mux  Inputs=2
  Out1 : Outport
  wires:
  Mux/1 -> D/1
  In1/1 -> Mux/1  "v_b"
  In2/1 -> Mux/2  "omega_b"
  D/1 -> Out1/1

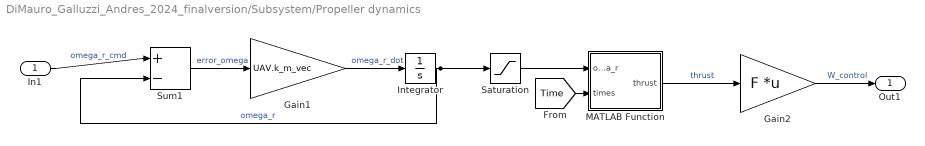
== system DiMauro_Galluzzi_Andres_2024_finalversion/Subsystem/Propeller dynamics ==
  In1 : Inport
  Gain1 : Gain  Gain=UAV.k_m_vec
  Gain2 : Gain  Gain=F  Multiplication=Matrix(K*u)
  Integrator : Integrator  InitialCondition=omega_r_0
  MATLAB Function : MATLAB Function  TreatAsAtomicUnit=on
  Saturation : Saturate  UpperLimit=UAV.Omega_max  LowerLimit=UAV.Omega_min
  Sum1 : Sum  Inputs=|+-
  Out1 : Outport
  wires:
  MATLAB Function/1(thrust) -> Gain2/1  "thrust"
  In1/1 -> Sum1/1  "omega_r_cmd"
  Integrator/1 -> Sum1/2, Saturation/1  "omega_r"
  Gain2/1 -> Out1/1  "W_control"
  Gain1/1 -> Integrator/1  "omega_r_dot"
  Saturation/1 -> MATLAB Function/1(omega_r)
  Sum1/1 -> Gain1/1  "error_omega"
  [Time] -> MATLAB Function/2(times)

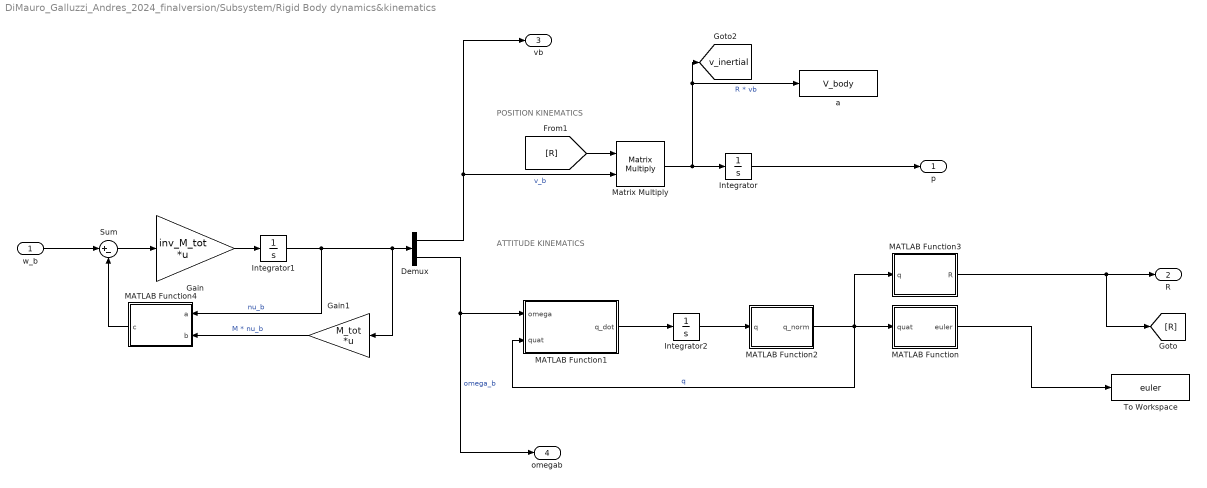
== system DiMauro_Galluzzi_Andres_2024_finalversion/Subsystem/Rigid Body dynamics&kinematics  ==
  note: ATTITUDE KINEMATICS
  note: POSITION KINEMATICS
  w_b : Inport
  Demux : Demux  Outputs=2
  Gain : Gain  Gain=inv_M_tot  Multiplication=Matrix(K*u)
  Gain1 : Gain  Gain=M_tot  Multiplication=Matrix(K*u)
  Integrator : Integrator  InitialCondition=p_0
  Integrator1 : Integrator  InitialCondition=[vb_0; omegab_0]
  Integrator2 : Integrator  InitialCondition=q_0
  MATLAB Function : MATLAB Function  TreatAsAtomicUnit=on
  MATLAB Function1 : MATLAB Function  TreatAsAtomicUnit=on
  MATLAB Function2 : MATLAB Function  TreatAsAtomicUnit=on
  MATLAB Function3 : MATLAB Function  TreatAsAtomicUnit=on
  MATLAB Function4 : MATLAB Function  TreatAsAtomicUnit=on
  Matrix Multiply : Product  Multiplication=Matrix(*)
  Sum : Sum  Inputs=|+-
  To Workspace : ToWorkspace  VariableName=euler  SaveFormat=Timeseries  SampleTime=-1
  a : ToWorkspace  VariableName=V_body  SaveFormat=Timeseries  SampleTime=-1
  p : Outport
  R : Outport  Port=2
  vb : Outport  Port=3
  omegab : Outport  Port=4
  tag scope: v_inertial=global
  wires:
  Integrator/1 -> p/1
  MATLAB Function1/1(q_dot) -> Integrator2/1
  MATLAB Function2/1(q_norm) -> MATLAB Function3/1(q), MATLAB Function1/2(quat), MATLAB Function/1(quat)  "q"
  MATLAB Function3/1(R) -> R/1, [R]
  Demux/1 -> Matrix Multiply/2, vb/1  "v_b"
  Integrator1/1 -> Demux/1, Gain1/1, MATLAB Function4/1(a)  "nu_b"
  Integrator2/1 -> MATLAB Function2/1(q)
  Matrix Multiply/1 -> [v_inertial], a/1, Integrator/1  "R * vb"
  MATLAB Function/1(euler) -> To Workspace/1
  [R] -> Matrix Multiply/1
  Gain/1 -> Integrator1/1
  Demux/2 -> omegab/1, MATLAB Function1/1(omega)  "omega_b"
  Gain1/1 -> MATLAB Function4/2(b)  "M * nu_b"
  Sum/1 -> Gain/1
  MATLAB Function4/1(c) -> Sum/2
  w_b/1 -> Sum/1

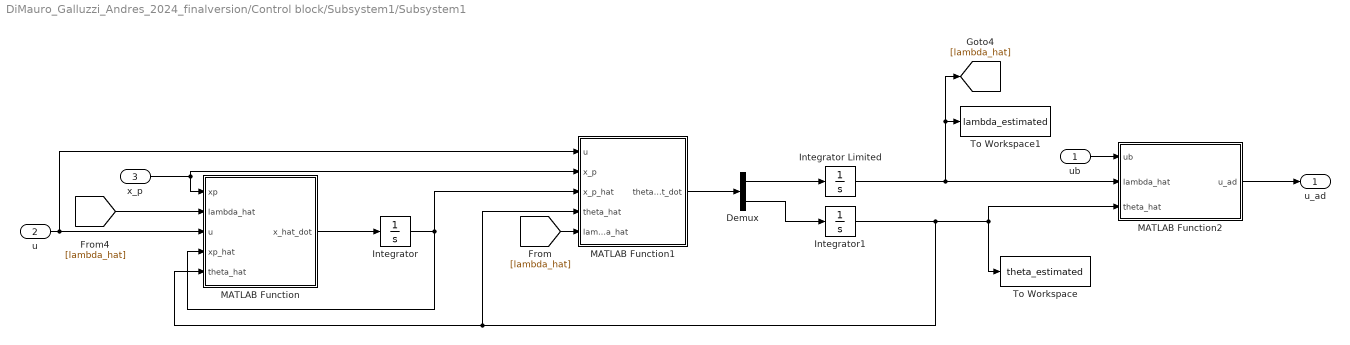
== system DiMauro_Galluzzi_Andres_2024_finalversion/Control block/Subsystem1/Subsystem1 ==
  ub : Inport
  u : Inport  Port=2
  x_p : Inport  Port=3
  Demux : Demux  Outputs=2
  Integrator : Integrator  InitialCondition=[0,0,0]'
  Integrator Limited : Integrator  InitialCondition=1/UAV.m*[1 1 1]'  LimitOutput=on  UpperSaturationLimit=1/UAV.m*[1 1 1]'  LowerSaturationLimit=[0 0 0]'
  Integrator1 : Integrator  InitialCondition=[0 0 0]'
  MATLAB Function : MATLAB Function  TreatAsAtomicUnit=on
  MATLAB Function1 : MATLAB Function  TreatAsAtomicUnit=on
  MATLAB Function2 : MATLAB Function  TreatAsAtomicUnit=on
  To Workspace : ToWorkspace  VariableName=theta_estimated  SaveFormat=Timeseries  SampleTime=-1
  To Workspace1 : ToWorkspace  VariableName=lambda_estimated  SaveFormat=Timeseries  SampleTime=-1
  u_ad : Outport
  wires:
  Integrator/1 -> MATLAB Function1/3(x_p_hat), MATLAB Function/4(xp_hat)
  [lambda_hat] -> MATLAB Function/2(lambda_hat)
  x_p/1 -> MATLAB Function/1(xp), MATLAB Function1/2(x_p)
  MATLAB Function2/1(u_ad) -> u_ad/1
  MATLAB Function/1(x_hat_dot) -> Integrator/1
  ub/1 -> MATLAB Function2/1(ub)
  MATLAB Function1/1(theta_a_hat_dot) -> Demux/1
  u/1 -> MATLAB Function/3(u), MATLAB Function1/1(u)
  Demux/1 -> Integrator Limited/1
  Integrator Limited/1 -> To Workspace1/1, [lambda_hat], MATLAB Function2/2(lambda_hat)
  Demux/2 -> Integrator1/1
  Integrator1/1 -> MATLAB Function1/4(theta_hat), MATLAB Function/5(theta_hat), To Workspace/1, MATLAB Function2/3(theta_hat)
  [lambda_hat] -> MATLAB Function1/5(lambda_hat)

== matlab function DiMauro_Galluzzi_Andres_2024_finalversion/Control block/Desired thrust normalization ==
  data: T_inertial output; f_c_inertial input
function T_inertial = norm(f_c_inertial)

T_inertial=norm(f_c_inertial); 
end

== matlab function DiMauro_Galluzzi_Andres_2024_finalversion/Control block/Attitude planner ==
  data: psi_d input; R_p output; f_c input
function R_p = attitude_planner(psi_d,f_c)

 k_p=f_c/norm(f_c); 
 h_p=[cos(psi_d), sin(psi_d), 0]';
 j_p=cross(k_p,h_p)/norm(cross(k_p,h_p)); 
 i_p=cross(j_p,k_p); 
 R_p=[i_p, j_p, k_p]; 
end

== matlab function DiMauro_Galluzzi_Andres_2024_finalversion/Control block/Attitude controller/e_R ==
  data: Rotm input; err_rot output; R_c input; k_R parameter
function err_rot = fcn(Rotm,R_c,k_R)
e_1 = [1 0 0]';
e_2 = [0 1 0]';
e_3 = [0 0 1]';
R_c_body = Rotm'*R_c; % transformation from desired to body frame coordinates

err_rot = k_R(1)*cross(R_c_body*e_1,e_1) + k_R(2)*cross(R_c_body*e_2,e_2) + k_R(3)*cross(R_c_body*e_3,e_3);

== matlab function DiMauro_Galluzzi_Andres_2024_finalversion/Control block/Control allocation ==
  data: tau input; Tc input; F parameter; k_f parameter; lambda_r_0 parameter; UAV parameter; omega_r_v output
function omega_r_v  = fcn(tau,Tc, F, k_f, lambda_r_0, UAV)

F_2=F(3:6,:);
F_2plus=F_2'/(F_2*F_2');
P_2=eye(6)-F_2plus*F_2;
F_1=[0 0 0 0; 0 0 0 0; eye(4)];


f_c=[0 0 Tc tau(1) tau(2) tau(3)]';
u_v= pinv(F_1)*f_c;

u_n=zeros(6,1);
u_cmd=F_2plus*u_v; % Minimum norm input

% To deal with saturation (does not take into account degradations)

lambda_r=lambda_r_0;
Tmin=lambda_r*k_f*UAV.Omega_min^2;
Tmax=lambda_r*k_f*UAV.Omega_max^2;


for i=1:6
    if u_cmd(i)<Tmin(i)
        u_n(i)=Tmin(i)-u_cmd(i);
    else 
        if u_cmd(i)>Tmax(i)
        u_n(i)=u_cmd(i)-Tmax(i);
        end
    end
end

u_cmd=F_2plus*u_v+P_2*u_n;

omega_r_v=zeros(length(u_cmd),1);
for i=1:length(u_cmd)
    omega_r_v(i)=sign(u_cmd(i))*sqrt(abs(u_cmd(i))./(lambda_r_0(i).*k_f));
end



end

== matlab function DiMauro_Galluzzi_Andres_2024_finalversion/Control block/Subsystem1/Subsystem1/MATLAB Function ==
  data: xp input; lambda_hat input; u input; x_hat_dot output; xp_hat input; Ap parameter; Bp parameter; g parameter; e parameter; L parameter; theta_hat input
function x_hat_dot = fcn(xp,lambda_hat,u,xp_hat, Ap, Bp,  g, e, L,theta_hat)

x_hat_dot=Ap*xp+Bp*(diag(lambda_hat)*u+eye(3)*theta_hat)-g*e+L*(xp-xp_hat);

== matlab function DiMauro_Galluzzi_Andres_2024_finalversion/Control block/Subsystem1/Subsystem1/MATLAB Function1 ==
  data: u input; theta_a_hat_dot output; x_p input; x_p_hat input; Gamma_a parameter; Bp parameter; theta_hat input; lambda_hat input
function theta_a_hat_dot=fcn(u,x_p,x_p_hat,Gamma_a, Bp,theta_hat,lambda_hat)
theta_a_hat=[lambda_hat;theta_hat];
phi_a=[diag(u) eye(3)]';

theta_a_hat_dot=Gamma_a*(phi_a*Bp'*(x_p-x_p_hat)-norm(Bp'*(x_p-x_p_hat))*theta_a_hat);

== matlab function DiMauro_Galluzzi_Andres_2024_finalversion/Control block/Subsystem1/Subsystem1/MATLAB Function2 ==
  data: ub input; u_ad output; lambda_hat input; theta_hat input
function u_ad  = fcn(ub,lambda_hat,theta_hat)

u_ad=(diag(1./lambda_hat)-eye(3))*ub-diag(1./lambda_hat)*eye(3)*theta_hat;

== matlab function DiMauro_Galluzzi_Andres_2024_finalversion/Control block/trajectory planner /MATLAB Function1 ==
  data: time input; p_d output; v_d output; a_d output; radius parameter; omega_t parameter; w_t parameter; psi_d output
function [p_d,v_d,a_d,psi_d] = trajectory_plan(time, radius, omega_t, w_t)


    % CIRCULAR TRAJECTORY
    p_d=[radius*cos(omega_t*time),radius*sin(omega_t*time),0]';
    v_d=[-radius*sin(omega_t*time)*omega_t,radius*cos(omega_t*time)*omega_t,0]';
    a_d=[-radius*cos(omega_t*time)*omega_t^2, -radius*sin(omega_t*time)*omega_t^2, 0]';
    psi_d=deg2rad(20); 


end

== matlab function DiMauro_Galluzzi_Andres_2024_finalversion/Control block/trajectory planner /MATLAB Function2 ==
  data: time input; p_d output; v_d output; a_d output; radius parameter; omega_t parameter; w_t parameter; psi_d output
function [p_d,v_d,a_d,psi_d] = trajectory_plan(time, radius, omega_t, w_t)


    %SETPOINT TRACKING
    p_d=[0,0,1]';
    v_d=[0 0 0]';
    a_d=[0 0 0]';
    psi_d=deg2rad(0);


end

== matlab function DiMauro_Galluzzi_Andres_2024_finalversion/Control block/trajectory planner /MATLAB Function3 ==
  data: time input; p_d output; v_d output; a_d output; radius parameter; omega_t parameter; w_t parameter; psi_d output
function [p_d,v_d,a_d,psi_d] = trajectory_plan(time, radius, omega_t, w_t)


    %LINEAR TRAJECTORY
    p_d=[0,time ,time]';
    v_d=[0 1 1]';
    a_d=[0 0 0]';
    psi_d=deg2rad(0);

end

== matlab function DiMauro_Galluzzi_Andres_2024_finalversion/Control block/trajectory planner /MATLAB Function4 ==
  data: time input; p_d output; v_d output; a_d output; radius parameter; omega_t parameter; w_t parameter; psi_d output
function [p_d,v_d,a_d,psi_d] = trajectory_plan(time, radius, omega_t, w_t)

    %QUADRATIC TRAJECTORY
    p_d=[2*time,0 ,0]';
    v_d=[2 0 0]';
    a_d=[0 0 0]';
    psi_d=deg2rad(0);

end

== matlab function DiMauro_Galluzzi_Andres_2024_finalversion/Control block/trajectory planner /MATLAB Function5 ==
  data: time input; p_d output; v_d output; a_d output; psi_d output
  function [p_d,v_d,a_d,psi_d] = trajectory_plan(time)
       persistent traj_data
       
       if isempty(traj_data)
           % Load trajectory data once
           loaded = load('trajectory_data.mat');
           traj_data = loaded.trajectory_data;
       end
       
       % Interpolate trajectory
       if time <= traj_data.time(1)
           idx = 1;
           p_d = traj_data.pd(idx, :)';
           v_d = traj_data.vd(idx, :)';
           a_d = traj_data.ad(idx, :)';
           psi_d = traj_data.psid(idx);
       elseif time >= traj_data.time(end)
           idx = length(traj_data.time);
           p_d = traj_data.pd(idx, :)';
           v_d = [0; 0; 0];
           a_d = [0; 0; 0];
           psi_d = traj_data.psid(idx);
       else
           p_d = interp1(traj_data.time, traj_data.pd, time)';
           v_d = interp1(traj_data.time, traj_data.vd, time)';
           a_d = interp1(traj_data.time, traj_data.ad, time)';
           psi_d = interp1(traj_data.time, traj_data.psid, time);
       end
   end

== matlab function DiMauro_Galluzzi_Andres_2024_finalversion/Subsystem/Rigid Body dynamics&kinematics /MATLAB Function1 ==
  data: omega input; quat input; q_dot output
 function q_dot = quat_kin(omega, quat)
%#codegen

eta = quat(1);
eps = quat(2:4);

W=[-eps';
   skew(eps) + eta*eye(3)];

q_dot = 0.5*W*omega;

end

function S=skew(s)
S=[0  -s(3)  s(2);
    s(3)   0 -s(1);
    -s(2)  s(1)  0];
end

== matlab function DiMauro_Galluzzi_Andres_2024_finalversion/Subsystem/Rigid Body dynamics&kinematics /MATLAB Function ==
  data: quat input; euler output
function euler = quatToEuler( quat )
%	Converts a quaternion vector to ZYX Euler angles (RPY)

euler = quat2eul(quat','ZYX');

end

== matlab function DiMauro_Galluzzi_Andres_2024_finalversion/Subsystem/Rigid Body dynamics&kinematics /MATLAB Function2 ==
  data: q input; q_norm output
function q_norm = quat_norm( q )

norm = sqrt( q(1)^2 + q(2)^2 + q(3)^2 + q(4)^2 );

q_norm = 1/norm * q;

== matlab function DiMauro_Galluzzi_Andres_2024_finalversion/Subsystem/Rigid Body dynamics&kinematics /MATLAB Function3 ==
  data: q input; R output
function R = fcn(q)

R = quat2rotm(q');

end

== matlab function DiMauro_Galluzzi_Andres_2024_finalversion/Subsystem/Rigid Body dynamics&kinematics /MATLAB Function4 ==
  data: a input; c output; b input
function c = cross_six(a,b)

a_v = a(1:3);
a_omega = a(4:6);

cross_six = [crossmat(a_omega), zeros(3,3);
             crossmat(a_v), crossmat(a_omega)] ;

c = cross_six*b;

end

function S=crossmat(s)
S=[0  -s(3)  s(2);
    s(3)   0 -s(1);
    -s(2)  s(1)  0];
end

== matlab function DiMauro_Galluzzi_Andres_2024_finalversion/Subsystem/Weight ==
  data: R input; w_g output; M_tot parameter; g parameter; e parameter
function w_g = fcn(R,M_tot,g,e)

m=M_tot(1,1);
S=M_tot(4:6,1:3);
w_g = g*[m*R'*e; S*R'*e];

== matlab function DiMauro_Galluzzi_Andres_2024_finalversion/Subsystem/Propeller dynamics/MATLAB Function ==
  data: omega_r input; thrust output; lambda_r_0 parameter; times input; k_f parameter; degrad_flag parameter
function thrust= thrust(omega_r,lambda_r_0, times, k_f,degrad_flag)
if degrad_flag==1
    lambda_r=lambda_r_0*(1-(0.4/500)*times);
else
    lambda_r=lambda_r_0;
end
thrust=lambda_r.*k_f.*omega_r.^2
end

== matlab function DiMauro_Galluzzi_Andres_2024_finalversion/Control block/trajectory planner /MATLAB Function ==
  data: time input; p_d output; v_d output; a_d output; radius parameter; omega_t parameter; w_t parameter; psi_d output
function [p_d,v_d,a_d,psi_d] = trajectory_plan(time, radius, omega_t, w_t)

    %SPIRAL TRAJECTORY
    p_d=[radius*cos(omega_t*time), radius*sin(omega_t*time), w_t*time]'; 
    v_d=[-radius*sin(omega_t*time)*omega_t, radius*cos(omega_t*time)*omega_t, w_t]'; 
    a_d=[-radius*cos(omega_t*time)*omega_t^2, -radius*sin(omega_t*time)*omega_t^2, 0]';
    psi_d=omega_t*time; 

end

== matlab function DiMauro_Galluzzi_Andres_2024_finalversion/Subsystem/MATLAB Function ==
  data: D input; y output; R input
function y = fcn(D,R)
d=D(1:3);
y=-R*d;
